simulink model "Demo_LQR_HSD_first"  (R2018b)
settings: Solver=ode1  StartTime=0.0  StopTime=30  FixedStep=0.001  RelTol=1e-3
undefined symbols (not defined in the file): K
settings Model: Creator=Lenovo  LastModifiedBy=24473
settings DataIOCC: LimitDataPoints=on  SaveFormat=Array
settings OptimizationCC: BlockReduction=off  BooleanDataType=off  LifeSpan=inf
settings DebuggingCC: SaveWithParameterizedLinksMsg=none  UnderspecifiedInitializationDetection=Classic  MergeDetectMultiDrivingBlocksExec=none  SignalResolutionControl=TryResolveAllWithWarning  SFUnexpectedBacktrackingDiag=warning  SFNoUnconditionalDefaultTransitionDiag=warning  SFExecutionAtInitializationDiag=none
settings HardwareCC: ProdBitPerPointer=32  ProdBitPerSizeT=32  ProdBitPerPtrDiffT=32  ProdLargestAtomicFloat=None  ProdIntDivRoundTo=Undefined  ProdEndianess=Unspecified  ProdWordSize=32  ProdHWDeviceType=32-bit Generic  TargetUnknown=on
settings ModelReferenceCC: PropagateSignalLabelsOutOfModel=off
settings SFSimCC: SimUseLocalCustomCode=off
settings RTWCC: RTWUseLocalCustomCode=off
settings CodeAppCC: StateflowObjectComments=on
settings GRTTargetCC: TargetLangStandard=C89/C90 (ANSI)  GeneratePreprocessorConditionals=Disable all
settings ConfigComp: CovMetricSettings=dw  CovHtmlReporting=on  CovSaveCumulativeToWorkspaceVar=on  CovSaveSingleToWorkspaceVar=on  CovExternalEMLEnable=off  CovSFcnEnable=off

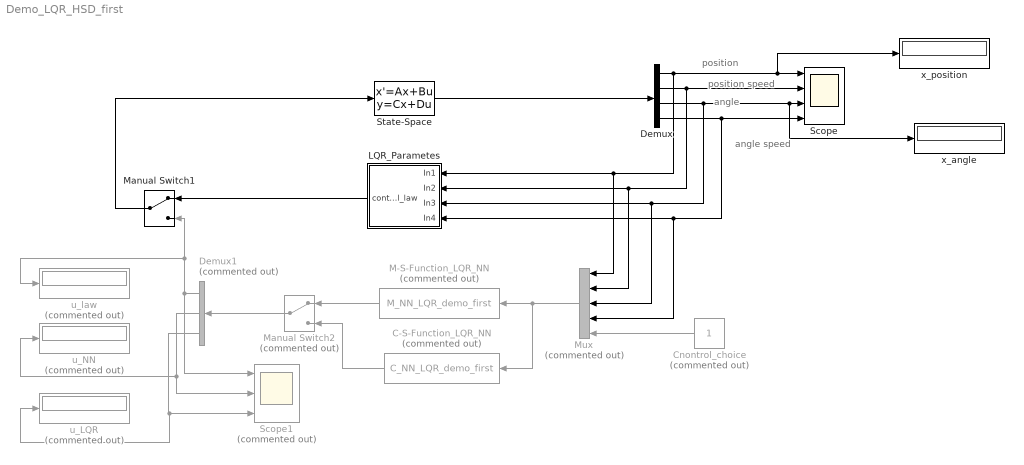
== system Demo_LQR_HSD_first ==
  note: angle speed
  note: angle
  note: position speed
  note: position
  C-S-Function_LQR_NN : S-Function  Commented=on  FunctionName=C_NN_LQR_demo_first  SFunctionDeploymentMode=off  EnableBusSupport=off
  Cnontrol_choice : Constant  Commented=on
  Demux : Demux
  Demux1 : Demux  Commented=on  Outputs=3
  LQR_Parametes : Subsystem
  M-S-Function_LQR_NN : S-Function  Commented=on  FunctionName=M_NN_LQR_demo_first  SFunctionDeploymentMode=off  EnableBusSupport=off
  Manual Switch1 : ManualSwitch
  Manual Switch2 : ManualSwitch  Commented=on
  Mux : Mux  Commented=on  Inputs=5
  Scope : Scope  NumInputPorts=4
  Scope1 : Scope  Commented=on  NumInputPorts=3
  State-Space : StateSpace  A=[0 1 0 0;0 -0.1164 1.2373 0;0 0 0 1;0 -0.7164 67.9221 0]  B=[0;1.4554;0;8.9546]  C=[1 0 0 0;0 1 0 0;0 0 1 0;0 0 0 1]  D=[0;0;0;0]  InitialCondition=[1;1;1;1]
  u_LQR : Display  Commented=on
  u_NN : Display  Commented=on
  u_law : Display  Commented=on
  x_angle : Display
  x_position : Display
  wires:
  State-Space/1 -> Demux/1
  Demux/1 -> LQR_Parametes/1(In1), Mux/1, x_position/1, Scope/1
  Demux/2 -> LQR_Parametes/2(In2), Mux/2, Scope/2
  Demux/4 -> LQR_Parametes/4(In4), Mux/4, Scope/4
  LQR_Parametes/1(control_law) -> Manual Switch1/1
  Mux/1 -> M-S-Function_LQR_NN/1, C-S-Function_LQR_NN/1
  Demux/3 -> LQR_Parametes/3(In3), Mux/3, x_angle/1, Scope/3
  Demux1/1 -> u_law/1, Manual Switch1/2, Scope1/1
  Demux1/2 -> Scope1/2, u_NN/1
  Demux1/3 -> u_LQR/1, Scope1/3
  Manual Switch1/1 -> State-Space/1
  Cnontrol_choice/1 -> Mux/5
  Manual Switch2/1 -> Demux1/1
  M-S-Function_LQR_NN/1 -> Manual Switch2/1
  C-S-Function_LQR_NN/1 -> Manual Switch2/2

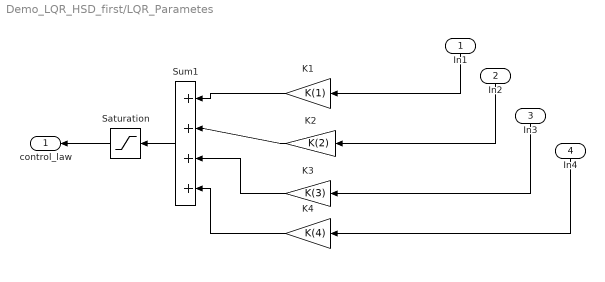
== system Demo_LQR_HSD_first/LQR_Parametes ==
  In1 : Inport
  In2 : Inport  Port=2
  In3 : Inport  Port=3
  In4 : Inport  Port=4
  K1 : Gain  Gain=K(1)
  K2 : Gain  Gain=K(2)
  K3 : Gain  Gain=K(3)
  K4 : Gain  Gain=K(4)
  Saturation : Saturate  UpperLimit=10  LowerLimit=-10
  Sum1 : Sum  Inputs=|++++
  control_law : Outport
  wires:
  In1/1 -> K1/1
  In3/1 -> K3/1
  In4/1 -> K4/1
  In2/1 -> K2/1
  K2/1 -> Sum1/2
  K1/1 -> Sum1/1
  K3/1 -> Sum1/3
  K4/1 -> Sum1/4
  Sum1/1 -> Saturation/1
  Saturation/1 -> control_law/1
